simulink model "qless_forgetting_factor_16x16"  (R2021a)
settings: Solver=FixedStepDiscrete  StartTime=0.0  StopTime=stoptime*inf  RelTol=1e-3
InitFcn:
  | qless_init_16chan_fi
undefined symbols (not defined in the file): fc, numArrayElements, physconst, srcAngles, sv, Ts
libraries: hdlsllib x137, commfilt2 x4, commrfcorlib x3, commsync2 x3, commrflib2 x2, commrandsrc3 x2, phasedtxrxlib x2, commdigbbndcpm2 x1, simulink x1, embreciprocals x1, commdigbbndpm3 x1
(part 7 of 22)

== system qless_forgetting_factor_16x16/MVDR_QLess_HDL/Complex Partial-Systolic Matrix Solve Using Q-less QR Decomposition with Forgetting Factor Manually Tiled n=16/Complex Q-less QR Forward Backward Substitute/Complex Burst Back Substitute with Matrix Output1/Reciprocal of the diagonal element/Positive Normalized Reciprocal HDL Optimized ==
  u : Inport
  validIn : Inport  Port=2
  Delay{,1..5} (6 alike) : Delay  DelayLength=1
  Positive Real CORDIC Reciprocal Kernel HDL Optimized : Subsystem  mask(Positive Real CORDIC Reciprocal Kernel HDL Optimized){}
      mask help: fixed:emblib:PositiveRealCORDICReciprocalKernelFullDescription
      mask Help: For internal use only. This feature is intentionally undocumented. Its behavior may change, or it may be removed in a future release.
      mask Display:
      | text(0.5,0.8,'1 \leq x < 2','texmode','on','HorizontalAlignment','center')
      | text(0.5,0.6,'y = 1/x','texmode','on','HorizontalAlignment','center')
      | text(0.5,0.4,'0.5 < y \leq 1','texmode','on','HorizontalAlignment','center')
      | text(0.5,0.2,'e = e_{in}','texmode','on','HorizontalAlignment','center')
  Positive Real Normalizer HDL Optimized : Subsystem  mask(Positive Real Normalizer HDL Optimized){}
      mask help: fixed:emblib:PositiveRealNormalizerFullDescription
      mask Help: For internal use only. This feature is intentionally undocumented. Its behavior may change, or it may be removed in a future release.
      mask Display:
      | text(0.5,0.7,'u > 0','texmode','on','HorizontalAlignment','center')
      | text(0.5,0.5,'x = 2^e u','texmode','on','HorizontalAlignment','center')
      | text(0.5,0.3,'1 \leq x < 2','texmode','on','HorizontalAlignment','center')
  Unit Delay Enabled Synchronous : hdlsllib/Discrete/Unit Delay Enabled Synchronous  InitialCondition=0.0  SampleTime=-1
      settings: SourceProductBaseCode=SL
  Unit Delay Enabled Synchronous1 : hdlsllib/Discrete/Unit Delay Enabled Synchronous  InitialCondition=0.0  SampleTime=-1
      settings: SourceProductBaseCode=SL
  y : Outport  VectorParamsAs1DForOutWhenUnconnected=off
  e : Outport  Port=2  VectorParamsAs1DForOutWhenUnconnected=off
  validOut : Outport  Port=3  VectorParamsAs1DForOutWhenUnconnected=off
  wires:
  Delay5/1 -> validOut/1
  Positive Real CORDIC Reciprocal Kernel HDL Optimized/2(e) -> Unit Delay Enabled Synchronous1/1
  Positive Real CORDIC Reciprocal Kernel HDL Optimized/1(y) -> Unit Delay Enabled Synchronous/1
  Delay4/1 -> Positive Real CORDIC Reciprocal Kernel HDL Optimized/3(validIn)
  Delay3/1 -> Positive Real CORDIC Reciprocal Kernel HDL Optimized/2(e_in)
  Delay2/1 -> Positive Real CORDIC Reciprocal Kernel HDL Optimized/1(x)
  Positive Real Normalizer HDL Optimized/3(validOut) -> Delay4/1
  Positive Real Normalizer HDL Optimized/2(e) -> Delay3/1
  Positive Real Normalizer HDL Optimized/1(x) -> Delay2/1
  Delay1/1 -> Positive Real Normalizer HDL Optimized/2(validIn)
  Delay/1 -> Positive Real Normalizer HDL Optimized/1(u)
  Positive Real CORDIC Reciprocal Kernel HDL Optimized/3(validOut) -> Unit Delay Enabled Synchronous/2, Unit Delay Enabled Synchronous1/2, Delay5/1
  Unit Delay Enabled Synchronous1/1 -> e/1
  Unit Delay Enabled Synchronous/1 -> y/1
  u/1 -> Delay/1
  validIn/1 -> Delay1/1

== system qless_forgetting_factor_16x16/MVDR_QLess_HDL/Complex Partial-Systolic Matrix Solve Using Q-less QR Decomposition with Forgetting Factor Manually Tiled n=16/Complex Q-less QR Forward Backward Substitute/Complex Burst Forward Substitute with Matrix Output/Forward substitute logic/Complex-Complex Multiply1 ==
  row : Inport
  multiplier : Inport  Port=2
  Add1 : Sum  Inputs=+-  OutDataTypeStr=Inherit: Same as first input
  Add2 : Sum  OutDataTypeStr=Inherit: Same as first input
  Complex to Real-Imag : ComplexToRealImag
  Complex to Real-Imag1 : ComplexToRealImag
  D1_1 : Delay  DelayLength=1
  D1_2 : Delay  DelayLength=1
  D4_{1..4} (4 alike) : Delay  DelayLength=1
  Product{1..4} (4 alike) : Product  OutDataTypeStr=Inherit: Same as first input
  Real-Imag to Complex : RealImagToComplex
  output : Outport  VectorParamsAs1DForOutWhenUnconnected=off
  wires:
  Add2/1 -> Real-Imag to Complex/2
  Add1/1 -> Real-Imag to Complex/1
  D4_4/1 -> Add2/2
  D4_2/1 -> Add1/2
  Product4/1 -> D4_4/1
  D4_3/1 -> Add2/1
  Product2/1 -> D4_2/1
  D4_1/1 -> Add1/1
  Product3/1 -> D4_3/1
  Product1/1 -> D4_1/1
  Complex to Real-Imag1/2 -> Product2/2, Product4/2  "D"
  Complex to Real-Imag/2 -> Product2/1, Product3/1  "B"
  Complex to Real-Imag1/1 -> Product1/2, Product3/2  "C"
  Complex to Real-Imag/1 -> Product1/1, Product4/1  "A"
  D1_2/1 -> Complex to Real-Imag1/1
  D1_1/1 -> Complex to Real-Imag/1
  Real-Imag to Complex/1 -> output/1
  row/1 -> D1_1/1
  multiplier/1 -> D1_2/1

== system qless_forgetting_factor_16x16/MVDR_QLess_HDL/Complex Partial-Systolic Matrix Solve Using Q-less QR Decomposition with Forgetting Factor Manually Tiled n=16/Complex Q-less QR Forward Backward Substitute/Complex Burst Forward Substitute with Matrix Output/Forward substitute logic/Complex-Real Multiply ==
  row : Inport
  multiplier : Inport  Port=2
  D1_1 : Delay  DelayLength=1
  D1_2 : Delay  DelayLength=1
  Delay : Delay  DelayLength=1
  Product : Product  OutDataTypeStr=Inherit: Same as first input
  output : Outport  VectorParamsAs1DForOutWhenUnconnected=off
  wires:
  D1_1/1 -> Product/1
  Product/1 -> Delay/1
  Delay/1 -> output/1
  D1_2/1 -> Product/2
  multiplier/1 -> D1_2/1
  row/1 -> D1_1/1

== system qless_forgetting_factor_16x16/MVDR_QLess_HDL/Complex Partial-Systolic Matrix Solve Using Q-less QR Decomposition with Forgetting Factor Manually Tiled n=16/Complex Q-less QR Forward Backward Substitute/Complex Burst Forward Substitute with Matrix Output/Forward substitute logic/Same Datatype ==
  Data : Inport
  Reference : Inport  Port=2
  Data Type Duplicate : DataTypeDuplicate
  DataOut : Outport  VectorParamsAs1DForOutWhenUnconnected=off
  wires:
  Reference/1 -> Data Type Duplicate/2
  Data/1 -> DataOut/1, Data Type Duplicate/1

== system qless_forgetting_factor_16x16/MVDR_QLess_HDL/Complex Partial-Systolic Matrix Solve Using Q-less QR Decomposition with Forgetting Factor Manually Tiled n=16/Complex Q-less QR Forward Backward Substitute/Complex Burst Forward Substitute with Matrix Output/Forward substitute logic/Same Datatype1 ==
  Data : Inport
  Reference : Inport  Port=2
  Data Type Duplicate : DataTypeDuplicate
  DataOut : Outport  VectorParamsAs1DForOutWhenUnconnected=off
  wires:
  Reference/1 -> Data Type Duplicate/2
  Data/1 -> DataOut/1, Data Type Duplicate/1

== system qless_forgetting_factor_16x16/MVDR_QLess_HDL/Complex Partial-Systolic Matrix Solve Using Q-less QR Decomposition with Forgetting Factor Manually Tiled n=16/Complex Q-less QR Forward Backward Substitute/Complex Burst Forward Substitute with Matrix Output/Forward substitute logic/Same Datatype2 ==
  Data : Inport
  Reference : Inport  Port=2
  Data Type Duplicate : DataTypeDuplicate
  DataOut : Outport  VectorParamsAs1DForOutWhenUnconnected=off
  wires:
  Reference/1 -> Data Type Duplicate/2
  Data/1 -> DataOut/1, Data Type Duplicate/1

== system qless_forgetting_factor_16x16/MVDR_QLess_HDL/Complex Partial-Systolic Matrix Solve Using Q-less QR Decomposition with Forgetting Factor Manually Tiled n=16/Complex Q-less QR Forward Backward Substitute/Complex Burst Forward Substitute with Matrix Output/Forward substitute logic/Same Datatype3 ==
  Data : Inport
  Reference : Inport  Port=2
  Data Type Duplicate : DataTypeDuplicate
  DataOut : Outport  VectorParamsAs1DForOutWhenUnconnected=off
  wires:
  Reference/1 -> Data Type Duplicate/2
  Data/1 -> DataOut/1, Data Type Duplicate/1

== system qless_forgetting_factor_16x16/MVDR_QLess_HDL/Complex Partial-Systolic Matrix Solve Using Q-less QR Decomposition with Forgetting Factor Manually Tiled n=16/Complex Q-less QR Forward Backward Substitute/Complex Burst Forward Substitute with Matrix Output/Forward substitute logic/Variable shift ==
  x : Inport
  shiftValue : Inport  Port=2
  MATLAB Function : MATLAB Function  TreatAsAtomicUnit=on
  y : Outport  VectorParamsAs1DForOutWhenUnconnected=off
  wires:
  shiftValue/1 -> MATLAB Function/2(shiftValue)
  MATLAB Function/1(y) -> y/1
  x/1 -> MATLAB Function/1(x)

== system qless_forgetting_factor_16x16/MVDR_QLess_HDL/Complex Partial-Systolic Matrix Solve Using Q-less QR Decomposition with Forgetting Factor Manually Tiled n=16/Complex Q-less QR Forward Backward Substitute/Complex Burst Forward Substitute with Matrix Output/Reciprocal of the diagonal element/Positive Normalized Reciprocal HDL Optimized ==
  u : Inport
  validIn : Inport  Port=2
  Delay{,1..5} (6 alike) : Delay  DelayLength=1
  Positive Real CORDIC Reciprocal Kernel HDL Optimized : Subsystem  mask(Positive Real CORDIC Reciprocal Kernel HDL Optimized){}
      mask help: fixed:emblib:PositiveRealCORDICReciprocalKernelFullDescription
      mask Help: For internal use only. This feature is intentionally undocumented. Its behavior may change, or it may be removed in a future release.
      mask Display:
      | text(0.5,0.8,'1 \leq x < 2','texmode','on','HorizontalAlignment','center')
      | text(0.5,0.6,'y = 1/x','texmode','on','HorizontalAlignment','center')
      | text(0.5,0.4,'0.5 < y \leq 1','texmode','on','HorizontalAlignment','center')
      | text(0.5,0.2,'e = e_{in}','texmode','on','HorizontalAlignment','center')
  Positive Real Normalizer HDL Optimized : Subsystem  mask(Positive Real Normalizer HDL Optimized){}
      mask help: fixed:emblib:PositiveRealNormalizerFullDescription
      mask Help: For internal use only. This feature is intentionally undocumented. Its behavior may change, or it may be removed in a future release.
      mask Display:
      | text(0.5,0.7,'u > 0','texmode','on','HorizontalAlignment','center')
      | text(0.5,0.5,'x = 2^e u','texmode','on','HorizontalAlignment','center')
      | text(0.5,0.3,'1 \leq x < 2','texmode','on','HorizontalAlignment','center')
  Unit Delay Enabled Synchronous : hdlsllib/Discrete/Unit Delay Enabled Synchronous  InitialCondition=0.0  SampleTime=-1
      settings: SourceProductBaseCode=SL
  Unit Delay Enabled Synchronous1 : hdlsllib/Discrete/Unit Delay Enabled Synchronous  InitialCondition=0.0  SampleTime=-1
      settings: SourceProductBaseCode=SL
  y : Outport  VectorParamsAs1DForOutWhenUnconnected=off
  e : Outport  Port=2  VectorParamsAs1DForOutWhenUnconnected=off
  validOut : Outport  Port=3  VectorParamsAs1DForOutWhenUnconnected=off
  wires:
  Delay5/1 -> validOut/1
  Positive Real CORDIC Reciprocal Kernel HDL Optimized/2(e) -> Unit Delay Enabled Synchronous1/1
  Positive Real CORDIC Reciprocal Kernel HDL Optimized/1(y) -> Unit Delay Enabled Synchronous/1
  Delay4/1 -> Positive Real CORDIC Reciprocal Kernel HDL Optimized/3(validIn)
  Delay3/1 -> Positive Real CORDIC Reciprocal Kernel HDL Optimized/2(e_in)
  Delay2/1 -> Positive Real CORDIC Reciprocal Kernel HDL Optimized/1(x)
  Positive Real Normalizer HDL Optimized/3(validOut) -> Delay4/1
  Positive Real Normalizer HDL Optimized/2(e) -> Delay3/1
  Positive Real Normalizer HDL Optimized/1(x) -> Delay2/1
  Delay1/1 -> Positive Real Normalizer HDL Optimized/2(validIn)
  Delay/1 -> Positive Real Normalizer HDL Optimized/1(u)
  Positive Real CORDIC Reciprocal Kernel HDL Optimized/3(validOut) -> Unit Delay Enabled Synchronous/2, Unit Delay Enabled Synchronous1/2, Delay5/1
  Unit Delay Enabled Synchronous1/1 -> e/1
  Unit Delay Enabled Synchronous/1 -> y/1
  u/1 -> Delay/1
  validIn/1 -> Delay1/1

== system qless_forgetting_factor_16x16/MVDR_QLess_HDL/Normalize Response/MVDR Weight Update/Inner Product/Element-wise complex product/HDL Complex Multiply ==
  note: Xilinx devices:
      | - Set D1 = 1 or 2 to trade off speed & FF resources
      | - Set D2-D5 = 1 to fully leverage DSP48 pipelines
      | - Use sync reset
      |
      | Intel FPGAs:
      | - Set D1 = 1 or 2 depending on device family
      | - Set D5 = 1; D2, D3, D4 = 0
      | - Use async reset
  In1 : Inport
  In2 : Inport  Port=2
  Add1 : Sum
  Add2 : Sum  Inputs=+-
  Add3 : Sum
  Add4 : Sum  Inputs=-+
  Add5 : Sum
  Complex to Real-Imag : ComplexToRealImag
  Complex to Real-Imag1 : ComplexToRealImag
  D1_1 : Delay  DelayLength=D1
  D1_2 : Delay  DelayLength=D1
  D2_{1..6} (6 alike) : Delay  DelayLength=D2
  D3_{1..5} (5 alike) : Delay  DelayLength=D3
  D4_1 : Delay  DelayLength=D4
  D4_2 : Delay  DelayLength=D4
  D4_3 : Delay  DelayLength=D4
  D5_1 : Delay  DelayLength=D5
  D5_2 : Delay  DelayLength=D5
  Product1 : Product  OutDataTypeStr=Inherit: Same as first input
  Product2 : Product  OutDataTypeStr=Inherit: Same as first input
  Product3 : Product  OutDataTypeStr=Inherit: Same as first input
  Real-Imag to Complex : RealImagToComplex
  Out1 : Outport  VectorParamsAs1DForOutWhenUnconnected=off
  wires:
  Real-Imag to Complex/1 -> Out1/1
  In2/1 -> D1_2/1
  Complex to Real-Imag1/1 -> Add3/1, D2_4/1  "C"
  Complex to Real-Imag1/2 -> Add3/2, D2_3/1  "D"
  Product1/1 -> D4_1/1  "X"
  Product2/1 -> D4_2/1  "Y"
  Product3/1 -> D3_5/1  "Z"
  Add4/1 -> D5_1/1
  Add5/1 -> D5_2/1
  D5_1/1 -> Real-Imag to Complex/1
  D5_2/1 -> Real-Imag to Complex/2
  D4_1/1 -> Add4/1
  D4_2/1 -> Add5/1
  D3_5/1 -> D4_3/1
  Add1/1 -> D3_1/1
  Add3/1 -> D2_6/1
  Add2/1 -> D3_3/1
  Complex to Real-Imag/1 -> D2_5/1, D2_1/1  "A"
  Complex to Real-Imag/2 -> D2_2/1  "B"
  D3_1/1 -> Product1/1
  D2_6/1 -> Product3/2
  D3_3/1 -> Product2/1
  D4_3/1 -> Add4/2, Add5/2
  D3_4/1 -> Product2/2
  D3_2/1 -> Product1/2
  D2_4/1 -> D3_4/1
  D2_3/1 -> D3_2/1
  D2_5/1 -> Product3/1
  D2_2/1 -> Add1/2, Add2/1
  D2_1/1 -> Add2/2, Add1/1
  In1/1 -> D1_1/1
  D1_1/1 -> Complex to Real-Imag/1
  D1_2/1 -> Complex to Real-Imag1/1

== system qless_forgetting_factor_16x16/MVDR_QLess_HDL/Complex Partial-Systolic Matrix Solve Using Q-less QR Decomposition with Forgetting Factor Manually Tiled n=16/Complex Partial-Systolic Q-less QR with Forgetting Factor/Complex Partial-Systolic Q-less QR with Forgetting Factor Manually tiled/Complex Partial-Systolic Q-less QR Decomposition with Forgetting Factor Section Constant pivot1/Complex Partial-Systolic Q-less QR Row Rotations/Complex Partial-Systolic Q-less QR CORDIC Row Rotation ==
  x : Inport
  y : Inport  Port=2
  validIn : Inport  Port=3
  restart : Inport  Port=4
  CORDIC QR Kernel : MATLAB Function  TreatAsAtomicUnit=on
  Delay{1..3,6} (4 alike) : Delay  DelayLength=1
  State Control : StateControl  StateControl=Synchronous
  Unit Delay Enabled Synchronous1 : hdlsllib/Discrete/Unit Delay Enabled Synchronous  InitialCondition=0.0  SampleTime=-1
      settings: SourceProductBaseCode=SL
  Unit Delay Enabled Synchronous4 : hdlsllib/Discrete/Unit Delay Enabled Synchronous  InitialCondition=0.0  SampleTime=-1
      settings: SourceProductBaseCode=SL
  xOut : Outport  VectorParamsAs1DForOutWhenUnconnected=off
  yOut : Outport  Port=2  VectorParamsAs1DForOutWhenUnconnected=off
  validOut : Outport  Port=3  VectorParamsAs1DForOutWhenUnconnected=off
  ready : Outport  Port=4  VectorParamsAs1DForOutWhenUnconnected=off
  wires:
  Delay3/1 -> validOut/1
  Unit Delay Enabled Synchronous1/1 -> yOut/1
  CORDIC QR Kernel/1(xOut) -> Unit Delay Enabled Synchronous4/1
  y/1 -> Delay2/1
  x/1 -> Delay1/1
  CORDIC QR Kernel/2(yOut) -> Unit Delay Enabled Synchronous1/1
  validIn/1 -> Delay6/1
  Unit Delay Enabled Synchronous4/1 -> xOut/1
  restart/1 -> CORDIC QR Kernel/4(restart)
  CORDIC QR Kernel/3(validOut) -> Delay3/1, Unit Delay Enabled Synchronous4/2, Unit Delay Enabled Synchronous1/2
  CORDIC QR Kernel/4(ready) -> ready/1
  Delay1/1 -> CORDIC QR Kernel/1(xIn)
  Delay2/1 -> CORDIC QR Kernel/2(yIn)
  Delay6/1 -> CORDIC QR Kernel/3(validIn)

== system qless_forgetting_factor_16x16/MVDR_QLess_HDL/Complex Partial-Systolic Matrix Solve Using Q-less QR Decomposition with Forgetting Factor Manually Tiled n=16/Complex Partial-Systolic Q-less QR with Forgetting Factor/Complex Partial-Systolic Q-less QR with Forgetting Factor Manually tiled/Complex Partial-Systolic Q-less QR Decomposition with Forgetting Factor Section Constant pivot1/Complex Partial-Systolic Q-less QR Row Rotations/Inverse CORDIC Gain1 ==
  u : Inport
  MATLAB Function : MATLAB Function  TreatAsAtomicUnit=on
  y : Outport  VectorParamsAs1DForOutWhenUnconnected=off
  wires:
  MATLAB Function/1(y) -> y/1
  u/1 -> MATLAB Function/1(u)

== system qless_forgetting_factor_16x16/MVDR_QLess_HDL/Complex Partial-Systolic Matrix Solve Using Q-less QR Decomposition with Forgetting Factor Manually Tiled n=16/Complex Partial-Systolic Q-less QR with Forgetting Factor/Complex Partial-Systolic Q-less QR with Forgetting Factor Manually tiled/Complex Partial-Systolic Q-less QR Decomposition with Forgetting Factor Section Constant pivot1/Complex Partial-Systolic Q-less QR Row Rotations/Inverse CORDIC Gain4 ==
  u : Inport
  MATLAB Function : MATLAB Function  TreatAsAtomicUnit=on
  y : Outport  VectorParamsAs1DForOutWhenUnconnected=off
  wires:
  MATLAB Function/1(y) -> y/1
  u/1 -> MATLAB Function/1(u)

== system qless_forgetting_factor_16x16/MVDR_QLess_HDL/Complex Partial-Systolic Matrix Solve Using Q-less QR Decomposition with Forgetting Factor Manually Tiled n=16/Complex Partial-Systolic Q-less QR with Forgetting Factor/Complex Partial-Systolic Q-less QR with Forgetting Factor Manually tiled/Complex Partial-Systolic Q-less QR Decomposition with Forgetting Factor Section Constant pivot1/Complex Partial-Systolic Q-less QR Row Rotations/Q-less QR Rotate First Element To Real1 ==
  x : Inport
  validIn : Inport  Port=2
  restart : Inport  Port=3
  Complex to Real-Imag : ComplexToRealImag
  Delay15 : Delay  DelayLength=1
  Delay9 : Delay  DelayLength=1
  Q-less QR Real Row Rotations : Subsystem  mask(QR Real Row Rotations){n=n, pivot=pivot}
      mask prompts: n "fixed:emblib:ColumnsInA"
      mask help: fixed:emblib:RowRotationsFullDescription
      mask DialogControl n Prompt: Number of columns in matrix A
  Real-Imag to Complex : RealImagToComplex
  State Control : StateControl  StateControl=Synchronous
  Unit Delay Enabled Synchronous1 : hdlsllib/Discrete/Unit Delay Enabled Synchronous  InitialCondition=0.0  SampleTime=-1
      settings: SourceProductBaseCode=SL
  Unit Delay Enabled Synchronous3 : hdlsllib/Discrete/Unit Delay Enabled Synchronous  InitialCondition=0.0  SampleTime=-1
      settings: SourceProductBaseCode=SL
  ValidIn to Ready Logic : Subsystem
  ValidIn to Ready Logic1 : Subsystem
  xOut : Outport  VectorParamsAs1DForOutWhenUnconnected=off
  validOut : Outport  Port=2  VectorParamsAs1DForOutWhenUnconnected=off
  ready : Outport  Port=3  VectorParamsAs1DForOutWhenUnconnected=off
  wires:
  Q-less QR Real Row Rotations/2(yOut) -> Real-Imag to Complex/2
  Q-less QR Real Row Rotations/1(xOut) -> Real-Imag to Complex/1
  Complex to Real-Imag/2 -> Q-less QR Real Row Rotations/2(y)
  Complex to Real-Imag/1 -> Q-less QR Real Row Rotations/1(x)
  restart/1 -> Q-less QR Real Row Rotations/4(restart)
  ValidIn to Ready Logic1/1(readyOut) -> ready/1
  ValidIn to Ready Logic/1(readyOut) -> ValidIn to Ready Logic1/1(readyIn)
  Q-less QR Real Row Rotations/4(ready) -> ValidIn to Ready Logic/1(readyIn)
  Q-less QR Real Row Rotations/3(validOut) -> Delay15/1, Unit Delay Enabled Synchronous3/2
  Delay9/1 -> ValidIn to Ready Logic/2(validIn), Q-less QR Real Row Rotations/3(validIn)
  x/1 -> Unit Delay Enabled Synchronous1/1
  validIn/1 -> ValidIn to Ready Logic1/2(validIn), Delay9/1, Unit Delay Enabled Synchronous1/2
  Delay15/1 -> validOut/1
  Unit Delay Enabled Synchronous1/1 -> Complex to Real-Imag/1
  Real-Imag to Complex/1 -> Unit Delay Enabled Synchronous3/1
  Unit Delay Enabled Synchronous3/1 -> xOut/1

== system qless_forgetting_factor_16x16/MVDR_QLess_HDL/Complex Partial-Systolic Matrix Solve Using Q-less QR Decomposition with Forgetting Factor Manually Tiled n=16/Complex Partial-Systolic Q-less QR with Forgetting Factor/Complex Partial-Systolic Q-less QR with Forgetting Factor Manually tiled/Complex Partial-Systolic Q-less QR Decomposition with Forgetting Factor Section Constant pivot1/Complex Partial-Systolic Q-less QR Row Rotations/Set Element To Zero1 ==
  u : Inport
  Set Element To Zero : MATLAB Function  TreatAsAtomicUnit=on
  y : Outport  VectorParamsAs1DForOutWhenUnconnected=off
  wires:
  Set Element To Zero/1(y) -> y/1
  u/1 -> Set Element To Zero/1(u)

== system qless_forgetting_factor_16x16/MVDR_QLess_HDL/Complex Partial-Systolic Matrix Solve Using Q-less QR Decomposition with Forgetting Factor Manually Tiled n=16/Complex Partial-Systolic Q-less QR with Forgetting Factor/Complex Partial-Systolic Q-less QR with Forgetting Factor Manually tiled/Complex Partial-Systolic Q-less QR Decomposition with Forgetting Factor Section Constant pivot1/Complex Partial-Systolic Q-less QR Row Rotations/ValidIn to Ready Logic ==
  readyIn : Inport
  validIn : Inport  Port=2
  AND : Logic  IconShape=distinctive  AllPortsSameDT=off  OutDataTypeStr=boolean
  NOT : Logic  Operator=NOT  IconShape=distinctive  AllPortsSameDT=off  OutDataTypeStr=boolean
  readyOut : Outport  VectorParamsAs1DForOutWhenUnconnected=off
  wires:
  validIn/1 -> NOT/1
  readyIn/1 -> AND/1
  AND/1 -> readyOut/1
  NOT/1 -> AND/2

== system qless_forgetting_factor_16x16/MVDR_QLess_HDL/Complex Partial-Systolic Matrix Solve Using Q-less QR Decomposition with Forgetting Factor Manually Tiled n=16/Complex Partial-Systolic Q-less QR with Forgetting Factor/Complex Partial-Systolic Q-less QR with Forgetting Factor Manually tiled/Complex Partial-Systolic Q-less QR Decomposition with Forgetting Factor Section Constant pivot1/Complex Partial-Systolic Q-less QR Row Rotations/ValidIn to Ready Logic1 ==
  readyIn : Inport
  validIn : Inport  Port=2
  AND : Logic  IconShape=distinctive  AllPortsSameDT=off  OutDataTypeStr=boolean
  NOT : Logic  Operator=NOT  IconShape=distinctive  AllPortsSameDT=off  OutDataTypeStr=boolean
  readyOut : Outport  VectorParamsAs1DForOutWhenUnconnected=off
  wires:
  validIn/1 -> NOT/1
  readyIn/1 -> AND/1
  AND/1 -> readyOut/1
  NOT/1 -> AND/2

== system qless_forgetting_factor_16x16/MVDR_QLess_HDL/Complex Partial-Systolic Matrix Solve Using Q-less QR Decomposition with Forgetting Factor Manually Tiled n=16/Complex Partial-Systolic Q-less QR with Forgetting Factor/Complex Partial-Systolic Q-less QR with Forgetting Factor Manually tiled/Complex Partial-Systolic Q-less QR Decomposition with Forgetting Factor Section Constant pivot10/Complex Partial-Systolic Q-less QR Row Rotations/Complex Partial-Systolic Q-less QR CORDIC Row Rotation ==
  x : Inport
  y : Inport  Port=2
  validIn : Inport  Port=3
  restart : Inport  Port=4
  CORDIC QR Kernel : MATLAB Function  TreatAsAtomicUnit=on
  Delay{1..3,6} (4 alike) : Delay  DelayLength=1
  State Control : StateControl  StateControl=Synchronous
  Unit Delay Enabled Synchronous1 : hdlsllib/Discrete/Unit Delay Enabled Synchronous  InitialCondition=0.0  SampleTime=-1
      settings: SourceProductBaseCode=SL
  Unit Delay Enabled Synchronous4 : hdlsllib/Discrete/Unit Delay Enabled Synchronous  InitialCondition=0.0  SampleTime=-1
      settings: SourceProductBaseCode=SL
  xOut : Outport  VectorParamsAs1DForOutWhenUnconnected=off
  yOut : Outport  Port=2  VectorParamsAs1DForOutWhenUnconnected=off
  validOut : Outport  Port=3  VectorParamsAs1DForOutWhenUnconnected=off
  ready : Outport  Port=4  VectorParamsAs1DForOutWhenUnconnected=off
  wires:
  Delay3/1 -> validOut/1
  Unit Delay Enabled Synchronous1/1 -> yOut/1
  CORDIC QR Kernel/1(xOut) -> Unit Delay Enabled Synchronous4/1
  y/1 -> Delay2/1
  x/1 -> Delay1/1
  CORDIC QR Kernel/2(yOut) -> Unit Delay Enabled Synchronous1/1
  validIn/1 -> Delay6/1
  Unit Delay Enabled Synchronous4/1 -> xOut/1
  restart/1 -> CORDIC QR Kernel/4(restart)
  CORDIC QR Kernel/3(validOut) -> Delay3/1, Unit Delay Enabled Synchronous4/2, Unit Delay Enabled Synchronous1/2
  CORDIC QR Kernel/4(ready) -> ready/1
  Delay1/1 -> CORDIC QR Kernel/1(xIn)
  Delay2/1 -> CORDIC QR Kernel/2(yIn)
  Delay6/1 -> CORDIC QR Kernel/3(validIn)

== system qless_forgetting_factor_16x16/MVDR_QLess_HDL/Complex Partial-Systolic Matrix Solve Using Q-less QR Decomposition with Forgetting Factor Manually Tiled n=16/Complex Partial-Systolic Q-less QR with Forgetting Factor/Complex Partial-Systolic Q-less QR with Forgetting Factor Manually tiled/Complex Partial-Systolic Q-less QR Decomposition with Forgetting Factor Section Constant pivot10/Complex Partial-Systolic Q-less QR Row Rotations/Inverse CORDIC Gain1 ==
  u : Inport
  MATLAB Function : MATLAB Function  TreatAsAtomicUnit=on
  y : Outport  VectorParamsAs1DForOutWhenUnconnected=off
  wires:
  MATLAB Function/1(y) -> y/1
  u/1 -> MATLAB Function/1(u)

== system qless_forgetting_factor_16x16/MVDR_QLess_HDL/Complex Partial-Systolic Matrix Solve Using Q-less QR Decomposition with Forgetting Factor Manually Tiled n=16/Complex Partial-Systolic Q-less QR with Forgetting Factor/Complex Partial-Systolic Q-less QR with Forgetting Factor Manually tiled/Complex Partial-Systolic Q-less QR Decomposition with Forgetting Factor Section Constant pivot10/Complex Partial-Systolic Q-less QR Row Rotations/Inverse CORDIC Gain4 ==
  u : Inport
  MATLAB Function : MATLAB Function  TreatAsAtomicUnit=on
  y : Outport  VectorParamsAs1DForOutWhenUnconnected=off
  wires:
  MATLAB Function/1(y) -> y/1
  u/1 -> MATLAB Function/1(u)

== system qless_forgetting_factor_16x16/MVDR_QLess_HDL/Complex Partial-Systolic Matrix Solve Using Q-less QR Decomposition with Forgetting Factor Manually Tiled n=16/Complex Partial-Systolic Q-less QR with Forgetting Factor/Complex Partial-Systolic Q-less QR with Forgetting Factor Manually tiled/Complex Partial-Systolic Q-less QR Decomposition with Forgetting Factor Section Constant pivot10/Complex Partial-Systolic Q-less QR Row Rotations/Q-less QR Rotate First Element To Real1 ==
  x : Inport
  validIn : Inport  Port=2
  restart : Inport  Port=3
  Complex to Real-Imag : ComplexToRealImag
  Delay15 : Delay  DelayLength=1
  Delay9 : Delay  DelayLength=1
  Q-less QR Real Row Rotations : Subsystem  mask(QR Real Row Rotations){n=n, pivot=pivot}
      mask prompts: n "fixed:emblib:ColumnsInA"
      mask help: fixed:emblib:RowRotationsFullDescription
      mask DialogControl n Prompt: Number of columns in matrix A
  Real-Imag to Complex : RealImagToComplex
  State Control : StateControl  StateControl=Synchronous
  Unit Delay Enabled Synchronous1 : hdlsllib/Discrete/Unit Delay Enabled Synchronous  InitialCondition=0.0  SampleTime=-1
      settings: SourceProductBaseCode=SL
  Unit Delay Enabled Synchronous3 : hdlsllib/Discrete/Unit Delay Enabled Synchronous  InitialCondition=0.0  SampleTime=-1
      settings: SourceProductBaseCode=SL
  ValidIn to Ready Logic : Subsystem
  ValidIn to Ready Logic1 : Subsystem
  xOut : Outport  VectorParamsAs1DForOutWhenUnconnected=off
  validOut : Outport  Port=2  VectorParamsAs1DForOutWhenUnconnected=off
  ready : Outport  Port=3  VectorParamsAs1DForOutWhenUnconnected=off
  wires:
  Q-less QR Real Row Rotations/2(yOut) -> Real-Imag to Complex/2
  Q-less QR Real Row Rotations/1(xOut) -> Real-Imag to Complex/1
  Complex to Real-Imag/2 -> Q-less QR Real Row Rotations/2(y)
  Complex to Real-Imag/1 -> Q-less QR Real Row Rotations/1(x)
  restart/1 -> Q-less QR Real Row Rotations/4(restart)
  ValidIn to Ready Logic1/1(readyOut) -> ready/1
  ValidIn to Ready Logic/1(readyOut) -> ValidIn to Ready Logic1/1(readyIn)
  Q-less QR Real Row Rotations/4(ready) -> ValidIn to Ready Logic/1(readyIn)
  Q-less QR Real Row Rotations/3(validOut) -> Delay15/1, Unit Delay Enabled Synchronous3/2
  Delay9/1 -> ValidIn to Ready Logic/2(validIn), Q-less QR Real Row Rotations/3(validIn)
  x/1 -> Unit Delay Enabled Synchronous1/1
  validIn/1 -> ValidIn to Ready Logic1/2(validIn), Delay9/1, Unit Delay Enabled Synchronous1/2
  Delay15/1 -> validOut/1
  Unit Delay Enabled Synchronous1/1 -> Complex to Real-Imag/1
  Real-Imag to Complex/1 -> Unit Delay Enabled Synchronous3/1
  Unit Delay Enabled Synchronous3/1 -> xOut/1

== system qless_forgetting_factor_16x16/MVDR_QLess_HDL/Complex Partial-Systolic Matrix Solve Using Q-less QR Decomposition with Forgetting Factor Manually Tiled n=16/Complex Partial-Systolic Q-less QR with Forgetting Factor/Complex Partial-Systolic Q-less QR with Forgetting Factor Manually tiled/Complex Partial-Systolic Q-less QR Decomposition with Forgetting Factor Section Constant pivot10/Complex Partial-Systolic Q-less QR Row Rotations/Set Element To Zero1 ==
  u : Inport
  Set Element To Zero : MATLAB Function  TreatAsAtomicUnit=on
  y : Outport  VectorParamsAs1DForOutWhenUnconnected=off
  wires:
  Set Element To Zero/1(y) -> y/1
  u/1 -> Set Element To Zero/1(u)

== system qless_forgetting_factor_16x16/MVDR_QLess_HDL/Complex Partial-Systolic Matrix Solve Using Q-less QR Decomposition with Forgetting Factor Manually Tiled n=16/Complex Partial-Systolic Q-less QR with Forgetting Factor/Complex Partial-Systolic Q-less QR with Forgetting Factor Manually tiled/Complex Partial-Systolic Q-less QR Decomposition with Forgetting Factor Section Constant pivot10/Complex Partial-Systolic Q-less QR Row Rotations/ValidIn to Ready Logic ==
  readyIn : Inport
  validIn : Inport  Port=2
  AND : Logic  IconShape=distinctive  AllPortsSameDT=off  OutDataTypeStr=boolean
  NOT : Logic  Operator=NOT  IconShape=distinctive  AllPortsSameDT=off  OutDataTypeStr=boolean
  readyOut : Outport  VectorParamsAs1DForOutWhenUnconnected=off
  wires:
  validIn/1 -> NOT/1
  readyIn/1 -> AND/1
  AND/1 -> readyOut/1
  NOT/1 -> AND/2

== system qless_forgetting_factor_16x16/MVDR_QLess_HDL/Complex Partial-Systolic Matrix Solve Using Q-less QR Decomposition with Forgetting Factor Manually Tiled n=16/Complex Partial-Systolic Q-less QR with Forgetting Factor/Complex Partial-Systolic Q-less QR with Forgetting Factor Manually tiled/Complex Partial-Systolic Q-less QR Decomposition with Forgetting Factor Section Constant pivot10/Complex Partial-Systolic Q-less QR Row Rotations/ValidIn to Ready Logic1 ==
  readyIn : Inport
  validIn : Inport  Port=2
  AND : Logic  IconShape=distinctive  AllPortsSameDT=off  OutDataTypeStr=boolean
  NOT : Logic  Operator=NOT  IconShape=distinctive  AllPortsSameDT=off  OutDataTypeStr=boolean
  readyOut : Outport  VectorParamsAs1DForOutWhenUnconnected=off
  wires:
  validIn/1 -> NOT/1
  readyIn/1 -> AND/1
  AND/1 -> readyOut/1
  NOT/1 -> AND/2

== system qless_forgetting_factor_16x16/MVDR_QLess_HDL/Complex Partial-Systolic Matrix Solve Using Q-less QR Decomposition with Forgetting Factor Manually Tiled n=16/Complex Partial-Systolic Q-less QR with Forgetting Factor/Complex Partial-Systolic Q-less QR with Forgetting Factor Manually tiled/Complex Partial-Systolic Q-less QR Decomposition with Forgetting Factor Section Constant pivot11/Complex Partial-Systolic Q-less QR Row Rotations/Complex Partial-Systolic Q-less QR CORDIC Row Rotation ==
  x : Inport
  y : Inport  Port=2
  validIn : Inport  Port=3
  restart : Inport  Port=4
  CORDIC QR Kernel : MATLAB Function  TreatAsAtomicUnit=on
  Delay{1..3,6} (4 alike) : Delay  DelayLength=1
  State Control : StateControl  StateControl=Synchronous
  Unit Delay Enabled Synchronous1 : hdlsllib/Discrete/Unit Delay Enabled Synchronous  InitialCondition=0.0  SampleTime=-1
      settings: SourceProductBaseCode=SL
  Unit Delay Enabled Synchronous4 : hdlsllib/Discrete/Unit Delay Enabled Synchronous  InitialCondition=0.0  SampleTime=-1
      settings: SourceProductBaseCode=SL
  xOut : Outport  VectorParamsAs1DForOutWhenUnconnected=off
  yOut : Outport  Port=2  VectorParamsAs1DForOutWhenUnconnected=off
  validOut : Outport  Port=3  VectorParamsAs1DForOutWhenUnconnected=off
  ready : Outport  Port=4  VectorParamsAs1DForOutWhenUnconnected=off
  wires:
  Delay3/1 -> validOut/1
  Unit Delay Enabled Synchronous1/1 -> yOut/1
  CORDIC QR Kernel/1(xOut) -> Unit Delay Enabled Synchronous4/1
  y/1 -> Delay2/1
  x/1 -> Delay1/1
  CORDIC QR Kernel/2(yOut) -> Unit Delay Enabled Synchronous1/1
  validIn/1 -> Delay6/1
  Unit Delay Enabled Synchronous4/1 -> xOut/1
  restart/1 -> CORDIC QR Kernel/4(restart)
  CORDIC QR Kernel/3(validOut) -> Delay3/1, Unit Delay Enabled Synchronous4/2, Unit Delay Enabled Synchronous1/2
  CORDIC QR Kernel/4(ready) -> ready/1
  Delay1/1 -> CORDIC QR Kernel/1(xIn)
  Delay2/1 -> CORDIC QR Kernel/2(yIn)
  Delay6/1 -> CORDIC QR Kernel/3(validIn)

== system qless_forgetting_factor_16x16/MVDR_QLess_HDL/Complex Partial-Systolic Matrix Solve Using Q-less QR Decomposition with Forgetting Factor Manually Tiled n=16/Complex Partial-Systolic Q-less QR with Forgetting Factor/Complex Partial-Systolic Q-less QR with Forgetting Factor Manually tiled/Complex Partial-Systolic Q-less QR Decomposition with Forgetting Factor Section Constant pivot11/Complex Partial-Systolic Q-less QR Row Rotations/Inverse CORDIC Gain1 ==
  u : Inport
  MATLAB Function : MATLAB Function  TreatAsAtomicUnit=on
  y : Outport  VectorParamsAs1DForOutWhenUnconnected=off
  wires:
  MATLAB Function/1(y) -> y/1
  u/1 -> MATLAB Function/1(u)

== system qless_forgetting_factor_16x16/MVDR_QLess_HDL/Complex Partial-Systolic Matrix Solve Using Q-less QR Decomposition with Forgetting Factor Manually Tiled n=16/Complex Partial-Systolic Q-less QR with Forgetting Factor/Complex Partial-Systolic Q-less QR with Forgetting Factor Manually tiled/Complex Partial-Systolic Q-less QR Decomposition with Forgetting Factor Section Constant pivot11/Complex Partial-Systolic Q-less QR Row Rotations/Inverse CORDIC Gain4 ==
  u : Inport
  MATLAB Function : MATLAB Function  TreatAsAtomicUnit=on
  y : Outport  VectorParamsAs1DForOutWhenUnconnected=off
  wires:
  MATLAB Function/1(y) -> y/1
  u/1 -> MATLAB Function/1(u)

== system qless_forgetting_factor_16x16/MVDR_QLess_HDL/Complex Partial-Systolic Matrix Solve Using Q-less QR Decomposition with Forgetting Factor Manually Tiled n=16/Complex Partial-Systolic Q-less QR with Forgetting Factor/Complex Partial-Systolic Q-less QR with Forgetting Factor Manually tiled/Complex Partial-Systolic Q-less QR Decomposition with Forgetting Factor Section Constant pivot11/Complex Partial-Systolic Q-less QR Row Rotations/Q-less QR Rotate First Element To Real1 ==
  x : Inport
  validIn : Inport  Port=2
  restart : Inport  Port=3
  Complex to Real-Imag : ComplexToRealImag
  Delay15 : Delay  DelayLength=1
  Delay9 : Delay  DelayLength=1
  Q-less QR Real Row Rotations : Subsystem  mask(QR Real Row Rotations){n=n, pivot=pivot}
      mask prompts: n "fixed:emblib:ColumnsInA"
      mask help: fixed:emblib:RowRotationsFullDescription
      mask DialogControl n Prompt: Number of columns in matrix A
  Real-Imag to Complex : RealImagToComplex
  State Control : StateControl  StateControl=Synchronous
  Unit Delay Enabled Synchronous1 : hdlsllib/Discrete/Unit Delay Enabled Synchronous  InitialCondition=0.0  SampleTime=-1
      settings: SourceProductBaseCode=SL
  Unit Delay Enabled Synchronous3 : hdlsllib/Discrete/Unit Delay Enabled Synchronous  InitialCondition=0.0  SampleTime=-1
      settings: SourceProductBaseCode=SL
  ValidIn to Ready Logic : Subsystem
  ValidIn to Ready Logic1 : Subsystem
  xOut : Outport  VectorParamsAs1DForOutWhenUnconnected=off
  validOut : Outport  Port=2  VectorParamsAs1DForOutWhenUnconnected=off
  ready : Outport  Port=3  VectorParamsAs1DForOutWhenUnconnected=off
  wires:
  Q-less QR Real Row Rotations/2(yOut) -> Real-Imag to Complex/2
  Q-less QR Real Row Rotations/1(xOut) -> Real-Imag to Complex/1
  Complex to Real-Imag/2 -> Q-less QR Real Row Rotations/2(y)
  Complex to Real-Imag/1 -> Q-less QR Real Row Rotations/1(x)
  restart/1 -> Q-less QR Real Row Rotations/4(restart)
  ValidIn to Ready Logic1/1(readyOut) -> ready/1
  ValidIn to Ready Logic/1(readyOut) -> ValidIn to Ready Logic1/1(readyIn)
  Q-less QR Real Row Rotations/4(ready) -> ValidIn to Ready Logic/1(readyIn)
  Q-less QR Real Row Rotations/3(validOut) -> Delay15/1, Unit Delay Enabled Synchronous3/2
  Delay9/1 -> ValidIn to Ready Logic/2(validIn), Q-less QR Real Row Rotations/3(validIn)
  x/1 -> Unit Delay Enabled Synchronous1/1
  validIn/1 -> ValidIn to Ready Logic1/2(validIn), Delay9/1, Unit Delay Enabled Synchronous1/2
  Delay15/1 -> validOut/1
  Unit Delay Enabled Synchronous1/1 -> Complex to Real-Imag/1
  Real-Imag to Complex/1 -> Unit Delay Enabled Synchronous3/1
  Unit Delay Enabled Synchronous3/1 -> xOut/1

== system qless_forgetting_factor_16x16/MVDR_QLess_HDL/Complex Partial-Systolic Matrix Solve Using Q-less QR Decomposition with Forgetting Factor Manually Tiled n=16/Complex Partial-Systolic Q-less QR with Forgetting Factor/Complex Partial-Systolic Q-less QR with Forgetting Factor Manually tiled/Complex Partial-Systolic Q-less QR Decomposition with Forgetting Factor Section Constant pivot11/Complex Partial-Systolic Q-less QR Row Rotations/Set Element To Zero1 ==
  u : Inport
  Set Element To Zero : MATLAB Function  TreatAsAtomicUnit=on
  y : Outport  VectorParamsAs1DForOutWhenUnconnected=off
  wires:
  Set Element To Zero/1(y) -> y/1
  u/1 -> Set Element To Zero/1(u)

== system qless_forgetting_factor_16x16/MVDR_QLess_HDL/Complex Partial-Systolic Matrix Solve Using Q-less QR Decomposition with Forgetting Factor Manually Tiled n=16/Complex Partial-Systolic Q-less QR with Forgetting Factor/Complex Partial-Systolic Q-less QR with Forgetting Factor Manually tiled/Complex Partial-Systolic Q-less QR Decomposition with Forgetting Factor Section Constant pivot11/Complex Partial-Systolic Q-less QR Row Rotations/ValidIn to Ready Logic ==
  readyIn : Inport
  validIn : Inport  Port=2
  AND : Logic  IconShape=distinctive  AllPortsSameDT=off  OutDataTypeStr=boolean
  NOT : Logic  Operator=NOT  IconShape=distinctive  AllPortsSameDT=off  OutDataTypeStr=boolean
  readyOut : Outport  VectorParamsAs1DForOutWhenUnconnected=off
  wires:
  validIn/1 -> NOT/1
  readyIn/1 -> AND/1
  AND/1 -> readyOut/1
  NOT/1 -> AND/2

== system qless_forgetting_factor_16x16/MVDR_QLess_HDL/Complex Partial-Systolic Matrix Solve Using Q-less QR Decomposition with Forgetting Factor Manually Tiled n=16/Complex Partial-Systolic Q-less QR with Forgetting Factor/Complex Partial-Systolic Q-less QR with Forgetting Factor Manually tiled/Complex Partial-Systolic Q-less QR Decomposition with Forgetting Factor Section Constant pivot11/Complex Partial-Systolic Q-less QR Row Rotations/ValidIn to Ready Logic1 ==
  readyIn : Inport
  validIn : Inport  Port=2
  AND : Logic  IconShape=distinctive  AllPortsSameDT=off  OutDataTypeStr=boolean
  NOT : Logic  Operator=NOT  IconShape=distinctive  AllPortsSameDT=off  OutDataTypeStr=boolean
  readyOut : Outport  VectorParamsAs1DForOutWhenUnconnected=off
  wires:
  validIn/1 -> NOT/1
  readyIn/1 -> AND/1
  AND/1 -> readyOut/1
  NOT/1 -> AND/2

== system qless_forgetting_factor_16x16/MVDR_QLess_HDL/Complex Partial-Systolic Matrix Solve Using Q-less QR Decomposition with Forgetting Factor Manually Tiled n=16/Complex Partial-Systolic Q-less QR with Forgetting Factor/Complex Partial-Systolic Q-less QR with Forgetting Factor Manually tiled/Complex Partial-Systolic Q-less QR Decomposition with Forgetting Factor Section Constant pivot12/Complex Partial-Systolic Q-less QR Row Rotations/Complex Partial-Systolic Q-less QR CORDIC Row Rotation ==
  x : Inport
  y : Inport  Port=2
  validIn : Inport  Port=3
  restart : Inport  Port=4
  CORDIC QR Kernel : MATLAB Function  TreatAsAtomicUnit=on
  Delay{1..3,6} (4 alike) : Delay  DelayLength=1
  State Control : StateControl  StateControl=Synchronous
  Unit Delay Enabled Synchronous1 : hdlsllib/Discrete/Unit Delay Enabled Synchronous  InitialCondition=0.0  SampleTime=-1
      settings: SourceProductBaseCode=SL
  Unit Delay Enabled Synchronous4 : hdlsllib/Discrete/Unit Delay Enabled Synchronous  InitialCondition=0.0  SampleTime=-1
      settings: SourceProductBaseCode=SL
  xOut : Outport  VectorParamsAs1DForOutWhenUnconnected=off
  yOut : Outport  Port=2  VectorParamsAs1DForOutWhenUnconnected=off
  validOut : Outport  Port=3  VectorParamsAs1DForOutWhenUnconnected=off
  ready : Outport  Port=4  VectorParamsAs1DForOutWhenUnconnected=off
  wires:
  Delay3/1 -> validOut/1
  Unit Delay Enabled Synchronous1/1 -> yOut/1
  CORDIC QR Kernel/1(xOut) -> Unit Delay Enabled Synchronous4/1
  y/1 -> Delay2/1
  x/1 -> Delay1/1
  CORDIC QR Kernel/2(yOut) -> Unit Delay Enabled Synchronous1/1
  validIn/1 -> Delay6/1
  Unit Delay Enabled Synchronous4/1 -> xOut/1
  restart/1 -> CORDIC QR Kernel/4(restart)
  CORDIC QR Kernel/3(validOut) -> Delay3/1, Unit Delay Enabled Synchronous4/2, Unit Delay Enabled Synchronous1/2
  CORDIC QR Kernel/4(ready) -> ready/1
  Delay1/1 -> CORDIC QR Kernel/1(xIn)
  Delay2/1 -> CORDIC QR Kernel/2(yIn)
  Delay6/1 -> CORDIC QR Kernel/3(validIn)

== system qless_forgetting_factor_16x16/MVDR_QLess_HDL/Complex Partial-Systolic Matrix Solve Using Q-less QR Decomposition with Forgetting Factor Manually Tiled n=16/Complex Partial-Systolic Q-less QR with Forgetting Factor/Complex Partial-Systolic Q-less QR with Forgetting Factor Manually tiled/Complex Partial-Systolic Q-less QR Decomposition with Forgetting Factor Section Constant pivot12/Complex Partial-Systolic Q-less QR Row Rotations/Inverse CORDIC Gain1 ==
  u : Inport
  MATLAB Function : MATLAB Function  TreatAsAtomicUnit=on
  y : Outport  VectorParamsAs1DForOutWhenUnconnected=off
  wires:
  MATLAB Function/1(y) -> y/1
  u/1 -> MATLAB Function/1(u)

== system qless_forgetting_factor_16x16/MVDR_QLess_HDL/Complex Partial-Systolic Matrix Solve Using Q-less QR Decomposition with Forgetting Factor Manually Tiled n=16/Complex Partial-Systolic Q-less QR with Forgetting Factor/Complex Partial-Systolic Q-less QR with Forgetting Factor Manually tiled/Complex Partial-Systolic Q-less QR Decomposition with Forgetting Factor Section Constant pivot12/Complex Partial-Systolic Q-less QR Row Rotations/Inverse CORDIC Gain4 ==
  u : Inport
  MATLAB Function : MATLAB Function  TreatAsAtomicUnit=on
  y : Outport  VectorParamsAs1DForOutWhenUnconnected=off
  wires:
  MATLAB Function/1(y) -> y/1
  u/1 -> MATLAB Function/1(u)

== system qless_forgetting_factor_16x16/MVDR_QLess_HDL/Complex Partial-Systolic Matrix Solve Using Q-less QR Decomposition with Forgetting Factor Manually Tiled n=16/Complex Partial-Systolic Q-less QR with Forgetting Factor/Complex Partial-Systolic Q-less QR with Forgetting Factor Manually tiled/Complex Partial-Systolic Q-less QR Decomposition with Forgetting Factor Section Constant pivot12/Complex Partial-Systolic Q-less QR Row Rotations/Q-less QR Rotate First Element To Real1 ==
  x : Inport
  validIn : Inport  Port=2
  restart : Inport  Port=3
  Complex to Real-Imag : ComplexToRealImag
  Delay15 : Delay  DelayLength=1
  Delay9 : Delay  DelayLength=1
  Q-less QR Real Row Rotations : Subsystem  mask(QR Real Row Rotations){n=n, pivot=pivot}
      mask prompts: n "fixed:emblib:ColumnsInA"
      mask help: fixed:emblib:RowRotationsFullDescription
      mask DialogControl n Prompt: Number of columns in matrix A
  Real-Imag to Complex : RealImagToComplex
  State Control : StateControl  StateControl=Synchronous
  Unit Delay Enabled Synchronous1 : hdlsllib/Discrete/Unit Delay Enabled Synchronous  InitialCondition=0.0  SampleTime=-1
      settings: SourceProductBaseCode=SL
  Unit Delay Enabled Synchronous3 : hdlsllib/Discrete/Unit Delay Enabled Synchronous  InitialCondition=0.0  SampleTime=-1
      settings: SourceProductBaseCode=SL
  ValidIn to Ready Logic : Subsystem
  ValidIn to Ready Logic1 : Subsystem
  xOut : Outport  VectorParamsAs1DForOutWhenUnconnected=off
  validOut : Outport  Port=2  VectorParamsAs1DForOutWhenUnconnected=off
  ready : Outport  Port=3  VectorParamsAs1DForOutWhenUnconnected=off
  wires:
  Q-less QR Real Row Rotations/2(yOut) -> Real-Imag to Complex/2
  Q-less QR Real Row Rotations/1(xOut) -> Real-Imag to Complex/1
  Complex to Real-Imag/2 -> Q-less QR Real Row Rotations/2(y)
  Complex to Real-Imag/1 -> Q-less QR Real Row Rotations/1(x)
  restart/1 -> Q-less QR Real Row Rotations/4(restart)
  ValidIn to Ready Logic1/1(readyOut) -> ready/1
  ValidIn to Ready Logic/1(readyOut) -> ValidIn to Ready Logic1/1(readyIn)
  Q-less QR Real Row Rotations/4(ready) -> ValidIn to Ready Logic/1(readyIn)
  Q-less QR Real Row Rotations/3(validOut) -> Delay15/1, Unit Delay Enabled Synchronous3/2
  Delay9/1 -> ValidIn to Ready Logic/2(validIn), Q-less QR Real Row Rotations/3(validIn)
  x/1 -> Unit Delay Enabled Synchronous1/1
  validIn/1 -> ValidIn to Ready Logic1/2(validIn), Delay9/1, Unit Delay Enabled Synchronous1/2
  Delay15/1 -> validOut/1
  Unit Delay Enabled Synchronous1/1 -> Complex to Real-Imag/1
  Real-Imag to Complex/1 -> Unit Delay Enabled Synchronous3/1
  Unit Delay Enabled Synchronous3/1 -> xOut/1

== system qless_forgetting_factor_16x16/MVDR_QLess_HDL/Complex Partial-Systolic Matrix Solve Using Q-less QR Decomposition with Forgetting Factor Manually Tiled n=16/Complex Partial-Systolic Q-less QR with Forgetting Factor/Complex Partial-Systolic Q-less QR with Forgetting Factor Manually tiled/Complex Partial-Systolic Q-less QR Decomposition with Forgetting Factor Section Constant pivot12/Complex Partial-Systolic Q-less QR Row Rotations/Set Element To Zero1 ==
  u : Inport
  Set Element To Zero : MATLAB Function  TreatAsAtomicUnit=on
  y : Outport  VectorParamsAs1DForOutWhenUnconnected=off
  wires:
  Set Element To Zero/1(y) -> y/1
  u/1 -> Set Element To Zero/1(u)

== system qless_forgetting_factor_16x16/MVDR_QLess_HDL/Complex Partial-Systolic Matrix Solve Using Q-less QR Decomposition with Forgetting Factor Manually Tiled n=16/Complex Partial-Systolic Q-less QR with Forgetting Factor/Complex Partial-Systolic Q-less QR with Forgetting Factor Manually tiled/Complex Partial-Systolic Q-less QR Decomposition with Forgetting Factor Section Constant pivot12/Complex Partial-Systolic Q-less QR Row Rotations/ValidIn to Ready Logic ==
  readyIn : Inport
  validIn : Inport  Port=2
  AND : Logic  IconShape=distinctive  AllPortsSameDT=off  OutDataTypeStr=boolean
  NOT : Logic  Operator=NOT  IconShape=distinctive  AllPortsSameDT=off  OutDataTypeStr=boolean
  readyOut : Outport  VectorParamsAs1DForOutWhenUnconnected=off
  wires:
  validIn/1 -> NOT/1
  readyIn/1 -> AND/1
  AND/1 -> readyOut/1
  NOT/1 -> AND/2

== system qless_forgetting_factor_16x16/MVDR_QLess_HDL/Complex Partial-Systolic Matrix Solve Using Q-less QR Decomposition with Forgetting Factor Manually Tiled n=16/Complex Partial-Systolic Q-less QR with Forgetting Factor/Complex Partial-Systolic Q-less QR with Forgetting Factor Manually tiled/Complex Partial-Systolic Q-less QR Decomposition with Forgetting Factor Section Constant pivot12/Complex Partial-Systolic Q-less QR Row Rotations/ValidIn to Ready Logic1 ==
  readyIn : Inport
  validIn : Inport  Port=2
  AND : Logic  IconShape=distinctive  AllPortsSameDT=off  OutDataTypeStr=boolean
  NOT : Logic  Operator=NOT  IconShape=distinctive  AllPortsSameDT=off  OutDataTypeStr=boolean
  readyOut : Outport  VectorParamsAs1DForOutWhenUnconnected=off
  wires:
  validIn/1 -> NOT/1
  readyIn/1 -> AND/1
  AND/1 -> readyOut/1
  NOT/1 -> AND/2

== system qless_forgetting_factor_16x16/MVDR_QLess_HDL/Complex Partial-Systolic Matrix Solve Using Q-less QR Decomposition with Forgetting Factor Manually Tiled n=16/Complex Partial-Systolic Q-less QR with Forgetting Factor/Complex Partial-Systolic Q-less QR with Forgetting Factor Manually tiled/Complex Partial-Systolic Q-less QR Decomposition with Forgetting Factor Section Constant pivot13/Complex Partial-Systolic Q-less QR Row Rotations/Complex Partial-Systolic Q-less QR CORDIC Row Rotation ==
  x : Inport
  y : Inport  Port=2
  validIn : Inport  Port=3
  restart : Inport  Port=4
  CORDIC QR Kernel : MATLAB Function  TreatAsAtomicUnit=on
  Delay{1..3,6} (4 alike) : Delay  DelayLength=1
  State Control : StateControl  StateControl=Synchronous
  Unit Delay Enabled Synchronous1 : hdlsllib/Discrete/Unit Delay Enabled Synchronous  InitialCondition=0.0  SampleTime=-1
      settings: SourceProductBaseCode=SL
  Unit Delay Enabled Synchronous4 : hdlsllib/Discrete/Unit Delay Enabled Synchronous  InitialCondition=0.0  SampleTime=-1
      settings: SourceProductBaseCode=SL
  xOut : Outport  VectorParamsAs1DForOutWhenUnconnected=off
  yOut : Outport  Port=2  VectorParamsAs1DForOutWhenUnconnected=off
  validOut : Outport  Port=3  VectorParamsAs1DForOutWhenUnconnected=off
  ready : Outport  Port=4  VectorParamsAs1DForOutWhenUnconnected=off
  wires:
  Delay3/1 -> validOut/1
  Unit Delay Enabled Synchronous1/1 -> yOut/1
  CORDIC QR Kernel/1(xOut) -> Unit Delay Enabled Synchronous4/1
  y/1 -> Delay2/1
  x/1 -> Delay1/1
  CORDIC QR Kernel/2(yOut) -> Unit Delay Enabled Synchronous1/1
  validIn/1 -> Delay6/1
  Unit Delay Enabled Synchronous4/1 -> xOut/1
  restart/1 -> CORDIC QR Kernel/4(restart)
  CORDIC QR Kernel/3(validOut) -> Delay3/1, Unit Delay Enabled Synchronous4/2, Unit Delay Enabled Synchronous1/2
  CORDIC QR Kernel/4(ready) -> ready/1
  Delay1/1 -> CORDIC QR Kernel/1(xIn)
  Delay2/1 -> CORDIC QR Kernel/2(yIn)
  Delay6/1 -> CORDIC QR Kernel/3(validIn)
